simulink model "QEKF"  (R2017b)
settings: Solver=FixedStepDiscrete  StartTime=0.0  StopTime=inf  RelTol=1e-3  EnableMultiTasking=on
InitFcn:
  | QEKF_InitFcn;
libraries: lib_StateEstimation x3
settings Model: xpc_rtwmakecfg_data=_xpcethercatlib_  ParamWorkspaceSource=ReferencedWorkspace  Creator=robot  LastModifiedBy=Ross Hartley
settings SolverCC: ConcurrentTasks=on
settings DataIOCC: SaveFormat=Array  SaveOutput=off  SignalLogging=off  DSMLogging=off  VisualizeSimOutput=off  SaveTime=off
settings OptimizationCC: DefaultParameterBehavior=Inlined  InlineInvariantSignals=on  LifeSpan=inf  SimCompilerOptimization=on  AccelVerboseBuild=on
settings DebuggingCC: AllowSymbolicDim=off  SFUnexpectedBacktrackingDiag=warning  SFNoUnconditionalDefaultTransitionDiag=warning  SFExecutionAtInitializationDiag=none
settings HardwareCC: ProdBitPerPointer=32  ProdBitPerSizeT=32  ProdBitPerPtrDiffT=32  ProdLargestAtomicFloat=None  ProdWordSize=32  ProdLongLongMode=on  ProdHWDeviceType=Generic->32-bit x86 compatible
settings ModelReferenceCC: ParallelModelReferenceMATLABWorkerInit=Copy Base Workspace  ModelReferenceNumInstancesAllowed=Single
settings SFSimCC: SimUserSources=$getFileList('QEKF_src')$  SimUserIncludeDirs=$getFileList('QEKF_includes')$  SFSimEcho=off
settings RTWCC: SystemTargetFile=slrt.tlc  TLCOptions=-axPCMaxOverloads=1000000000 -axPCMaxOverloadLen=1000000000  TemplateMakefile=slrt_default_tmf  Description=Simulink Real-Time  RTWUseSimCustomCode=on  CustomInclude=$getFileList('QEKF_includes')$  CustomSource=$getFileList('QEKF_src')$  CodeExecutionProfiling=on  RTWCompilerOptimization=on
settings CodeAppCC: GenerateComments=off  MaxIdLength=128  SimulinkBlockComments=off
settings SimulinkRealTimeCC: ExtMode=off
settings ConfigComp: CovMetricSettings=dw  CovHtmlReporting=on  CovSaveCumulativeToWorkspaceVar=on  CovSaveSingleToWorkspaceVar=on  CovExternalEMLEnable=off

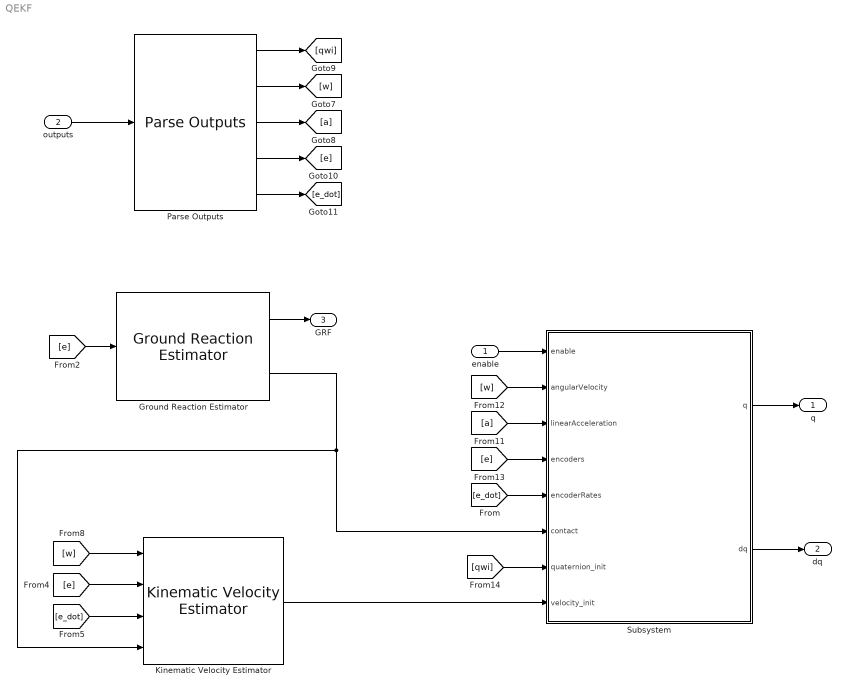
== system QEKF ==
  enable : Inport  BusOutputAsStruct=on
  outputs : Inport  Port=2  OutDataTypeStr=Bus: CassieOutBus  BusOutputAsStruct=on
  Ground Reaction Estimator : lib_StateEstimation/Ground Reaction Estimator
  Kinematic Velocity Estimator : lib_StateEstimation/Kinematic Velocity Estimator
  Parse Outputs : lib_StateEstimation/Parse Outputs
  Subsystem : Subsystem
  q : Outport
  dq : Outport  Port=2
  GRF : Outport  Port=3
  wires:
  enable/1 -> Subsystem/1(enable)
  [w] -> Subsystem/2(angularVelocity)
  [a] -> Subsystem/3(linearAcceleration)
  [e] -> Subsystem/4(encoders)
  Ground Reaction Estimator/2 -> Subsystem/6(contact), Kinematic Velocity Estimator/4
  Subsystem/1(q) -> q/1
  Subsystem/2(dq) -> dq/1
  Parse Outputs/1 -> [qwi]
  [w] -> Kinematic Velocity Estimator/1
  Kinematic Velocity Estimator/1 -> Subsystem/8(velocity_init)
  Parse Outputs/2 -> [w]
  [e] -> Kinematic Velocity Estimator/2
  outputs/1 -> Parse Outputs/1
  Parse Outputs/5 -> [e_dot]
  [e] -> Ground Reaction Estimator/1
  Ground Reaction Estimator/1 -> GRF/1
  [e_dot] -> Kinematic Velocity Estimator/3
  Parse Outputs/3 -> [a]
  Parse Outputs/4 -> [e]
  [qwi] -> Subsystem/7(quaternion_init)
  [e_dot] -> Subsystem/5(encoderRates)

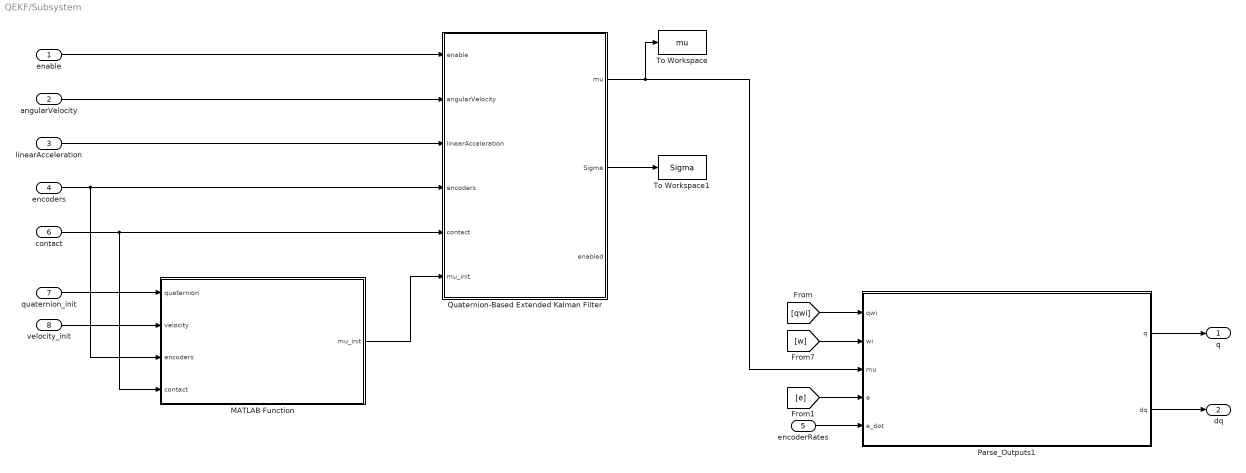
== system QEKF/Subsystem ==
  enable : Inport
  angularVelocity : Inport  Port=2
  linearAcceleration : Inport  Port=3
  encoders : Inport  Port=4
  encoderRates : Inport  Port=5
  contact : Inport  Port=6
  quaternion_init : Inport  Port=7
  velocity_init : Inport  Port=8
  MATLAB Function : MATLAB Function  TreatAsAtomicUnit=on
  Parse_Outputs1 : MATLAB Function  TreatAsAtomicUnit=on
  Quaternion-Based Extended Kalman Filter : Subsystem
  To Workspace : ToWorkspace  VariableName=mu  SaveFormat=Timeseries  SampleTime=-1
  To Workspace1 : ToWorkspace  VariableName=Sigma  SaveFormat=Timeseries  SampleTime=-1
  q : Outport
  dq : Outport  Port=2
  wires:
  Parse_Outputs1/2(dq) -> dq/1
  [e] -> Parse_Outputs1/4(e)
  [qwi] -> Parse_Outputs1/1(qwi)
  Parse_Outputs1/1(q) -> q/1
  encoderRates/1 -> Parse_Outputs1/5(e_dot)
  enable/1 -> Quaternion-Based Extended Kalman Filter/1(enable)
  angularVelocity/1 -> Quaternion-Based Extended Kalman Filter/2(angularVelocity)
  linearAcceleration/1 -> Quaternion-Based Extended Kalman Filter/3(linearAcceleration)
  Quaternion-Based Extended Kalman Filter/1(mu) -> Parse_Outputs1/3(mu), To Workspace/1
  Quaternion-Based Extended Kalman Filter/2(Sigma) -> To Workspace1/1
  [w] -> Parse_Outputs1/2(wi)
  MATLAB Function/1(mu_init) -> Quaternion-Based Extended Kalman Filter/6(mu_init)
  quaternion_init/1 -> MATLAB Function/1(quaternion)
  encoders/1 -> MATLAB Function/3(encoders), Quaternion-Based Extended Kalman Filter/4(encoders)
  contact/1 -> MATLAB Function/4(contact), Quaternion-Based Extended Kalman Filter/5(contact)
  velocity_init/1 -> MATLAB Function/2(velocity)

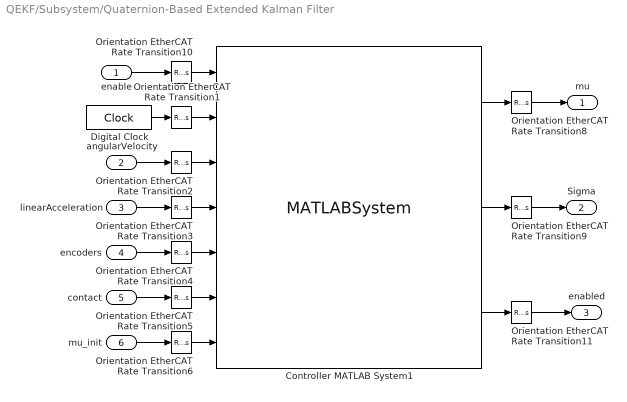
== system QEKF/Subsystem/Quaternion-Based Extended Kalman Filter ==
  enable : Inport
  angularVelocity : Inport  Port=2
  linearAcceleration : Inport  Port=3
  encoders : Inport  Port=4
  contact : Inport  Port=5
  mu_init : Inport  Port=6
  Controller MATLAB System1 : MATLABSystem  System=QuaternionEKF  static_bias_initialization=true  ekf_update_enabled=true  enable_bias_estimation=true  gyro_noise_std=0.1*ones( 3, 1 )  gyro_bias_noise_std=0.1*ones( 3, 1 )  accel_noise_std=0.1*ones( 3, 1 )  accel_bias_noise_std=0.1*ones( 3, 1 )  contact_noise_std=0.1*ones( 3, 1 )  encoder_noise_std=0.1*ones( 14, 1 )  gyro_bias_init=zeros( 3, 1 )  accel_bias_init=zeros( 3, 1 )  prior_base_pose_std=0.1*ones( 6, 1 )  prior_base_velocity_std=0.1*ones( 3, 1 )  prior_contact_position_std=0.1*ones( 3, 1 )  prior_gyro_bias_std=0.1*ones( 3, 1 )  prior_accel_bias_std=0.1*ones( 3, 1 )  prior_forward_kinematics_std=0.1*ones( 3, 1 )  SimulateUsing=Code generation
      mask Type: QuaternionEKF
      mask Display:
      | disp('QuaternionEKF');
      | port_label('input',1,'enable');
      | port_label('input',2,'t');
      | port_label('input',3,'w');
      | port_label('input',4,'a');
      | port_label('input',5,'encoders');
      | port_label('input',6,'contact');
      | port_label('input',7,'mu_init');
      | port_label('output',1,'mu');
      | port_label('output',2,'Sigma');
      | port_label('output',3,'enabled');
  Digital Clock : DigitalClock  SampleTime=-1
  Orientation EtherCAT Rate Transition{1..6,10} (7 alike) : RateTransition  Deterministic=off  OutPortSampleTime=EKF_SampleTime
  Orientation EtherCAT Rate Transition11 : RateTransition  Deterministic=off  OutPortSampleTime=0.0005
  Orientation EtherCAT Rate Transition8 : RateTransition  Deterministic=off  OutPortSampleTime=0.0005
  Orientation EtherCAT Rate Transition9 : RateTransition  Deterministic=off  OutPortSampleTime=0.0005
  mu : Outport
  Sigma : Outport  Port=2
  enabled : Outport  Port=3
  wires:
  angularVelocity/1 -> Orientation EtherCAT Rate Transition2/1
  Orientation EtherCAT Rate Transition4/1 -> Controller MATLAB System1/5
  Orientation EtherCAT Rate Transition10/1 -> Controller MATLAB System1/1
  Orientation EtherCAT Rate Transition11/1 -> enabled/1
  Controller MATLAB System1/1 -> Orientation EtherCAT Rate Transition8/1
  Orientation EtherCAT Rate Transition5/1 -> Controller MATLAB System1/6
  Orientation EtherCAT Rate Transition8/1 -> mu/1
  Orientation EtherCAT Rate Transition2/1 -> Controller MATLAB System1/3
  Orientation EtherCAT Rate Transition9/1 -> Sigma/1
  enable/1 -> Orientation EtherCAT Rate Transition10/1
  mu_init/1 -> Orientation EtherCAT Rate Transition6/1
  Controller MATLAB System1/3 -> Orientation EtherCAT Rate Transition11/1
  Digital Clock/1 -> Orientation EtherCAT Rate Transition1/1
  Controller MATLAB System1/2 -> Orientation EtherCAT Rate Transition9/1
  Orientation EtherCAT Rate Transition1/1 -> Controller MATLAB System1/2
  Orientation EtherCAT Rate Transition3/1 -> Controller MATLAB System1/4
  Orientation EtherCAT Rate Transition6/1 -> Controller MATLAB System1/7
  encoders/1 -> Orientation EtherCAT Rate Transition4/1
  contact/1 -> Orientation EtherCAT Rate Transition5/1
  linearAcceleration/1 -> Orientation EtherCAT Rate Transition3/1

== matlab function QEKF/Subsystem/Parse_Outputs1 ==
  data: q output; qwi input; wi input; dq output; mu input; e input; e_dot input
function [q, dq] = Contruct_State(qwi, wi, mu, e, e_dot)   
%   Author: Ross Hartley 
%   Date:   7/03/2017
%

% Compute Euler angles and rates 
Q = Quaternion(qwi);
qq = Q.getEulerAngles();
dqq = Angles.AngularVelocity_to_EulerRates(qq, wi);

% Construct State Vector
q = [mu(1:3); qq; e];
dq = [u(4:6); dqq; e_dot];

end

== matlab function QEKF/Subsystem/MATLAB Function ==
  data: quaternion input; velocity input; mu_init output; encoders input; contact input
function mu_init = InitialStateEstimate(quaternion, velocity, encoders, contact)

% R = Angles.Quaternion_to_Rotation(quaternion);
Q = Quaternion(quaternion);
R = Q.getRotation().getValue();
p = zeros(3,1); 
v = R*velocity;
pR = p_VectorNav_to_RightToeBottom(encoders);
pL = p_VectorNav_to_LeftToeBottom(encoders);

if contact(1) == 1
    % Initialize with left foot at 0
    p = -R * pL; % {W}_p_{WL}
elseif contact(2) == 1
    % Initialize with right foot at 0
    p = -R * pR; % {W}_p_{WR}
end

% Initial foot positions
dR = p + R * pR; % {W}_p_{WR}
dL = p + R * pL; % {W}_p_{WL}

% Construct Initial State
mu_init = [R, v, p, dR, dL; 0,0,0,1,0,0,0; 0,0,0,0,1,0,0; 0,0,0,0,0,1,0; 0,0,0,0,0,0,1];

end
